simulink model "plant"  (R2021b)
settings: Solver=FixedStepAuto  StartTime=0.0  StopTime=10.0  RelTol=1e-3
settings Model: Creator=DAUIN-Win10  LastModifiedBy=sagai

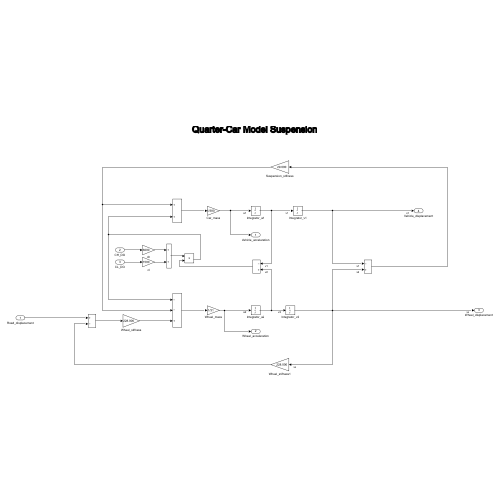
[thumbnail: Simulink's stored preview of the top-level diagram]
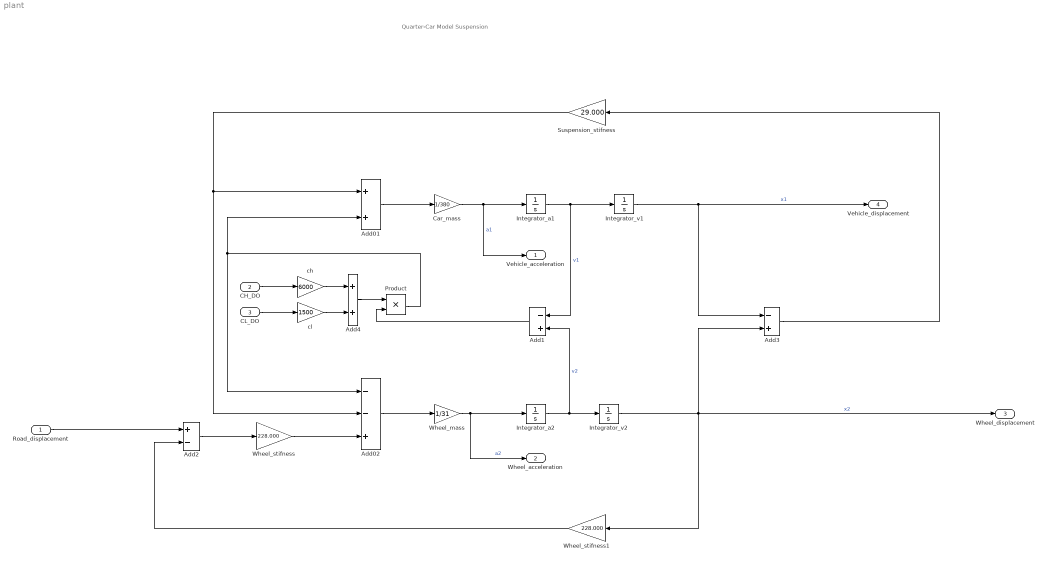
== system plant ==
  note: Quarter-Car Model Suspension
  Road_displacement : Inport
  CH_DO : Inport  Port=2  OutDataTypeStr=boolean
  CL_DO : Inport  Port=3  OutDataTypeStr=boolean
  Add01 : Sum
  Add02 : Sum  Inputs=--+
  Add1 : Sum  Inputs=-+
  Add2 : Sum  Inputs=+-
  Add3 : Sum  Inputs=-+
  Add4 : Sum  AccumDataTypeStr=double
  Car_mass : Gain  Gain=1/380
  Integrator_a1 : Integrator
  Integrator_a2 : Integrator
  Integrator_v1 : Integrator
  Integrator_v2 : Integrator
  Product : Product
  Suspension_stifness : Gain  Gain=29.000
  Wheel_mass : Gain  Gain=1/31
  Wheel_stifness : Gain  Gain=228.000
  Wheel_stifness1 : Gain  Gain=228.000
  ch : Gain  Gain=6000  OutDataTypeStr=double
  cl : Gain  Gain=1500  OutDataTypeStr=double
  Vehicle_acceleration : Outport
  Wheel_acceleration : Outport  Port=2
  Wheel_displacement : Outport  Port=3
  Vehicle_displacement : Outport  Port=4
  wires:
  Integrator_v1/1 -> Add3/1, Vehicle_displacement/1  "x1"
  Wheel_stifness1/1 -> Add2/2
  Road_displacement/1 -> Add2/1
  Add3/1 -> Suspension_stifness/1
  Suspension_stifness/1 -> Add02/2, Add01/1
  Product/1 -> Add02/1, Add01/2
  Add1/1 -> Product/2
  Integrator_v2/1 -> Wheel_stifness1/1, Wheel_displacement/1, Add3/2  "x2"
  Add2/1 -> Wheel_stifness/1
  Integrator_a1/1 -> Integrator_v1/1, Add1/1  "v1"
  Add01/1 -> Car_mass/1
  Add4/1 -> Product/1
  Add02/1 -> Wheel_mass/1
  Wheel_mass/1 -> Integrator_a2/1, Wheel_acceleration/1  "a2"
  Wheel_stifness/1 -> Add02/3
  Integrator_a2/1 -> Integrator_v2/1, Add1/2  "v2"
  Car_mass/1 -> Integrator_a1/1, Vehicle_acceleration/1  "a1"
  CL_DO/1 -> cl/1
  CH_DO/1 -> ch/1
  ch/1 -> Add4/1
  cl/1 -> Add4/2
